simulink model "dec_2_3"  (R2013b)
settings: Solver=ode45  StartTime=0.0  StopTime=10000  RelTol=1e-3
undefined symbols (not defined in the file or in its folder): pfb_coeff_gen_calc, xlfda_numerator, xlipgetpartsetting
libraries: xbsIndex_r4 x2069, casper_library_delays x25, dspsigops x16, casper_library_misc x11, simulink x1, xps_library x1
(part 3 of 19)

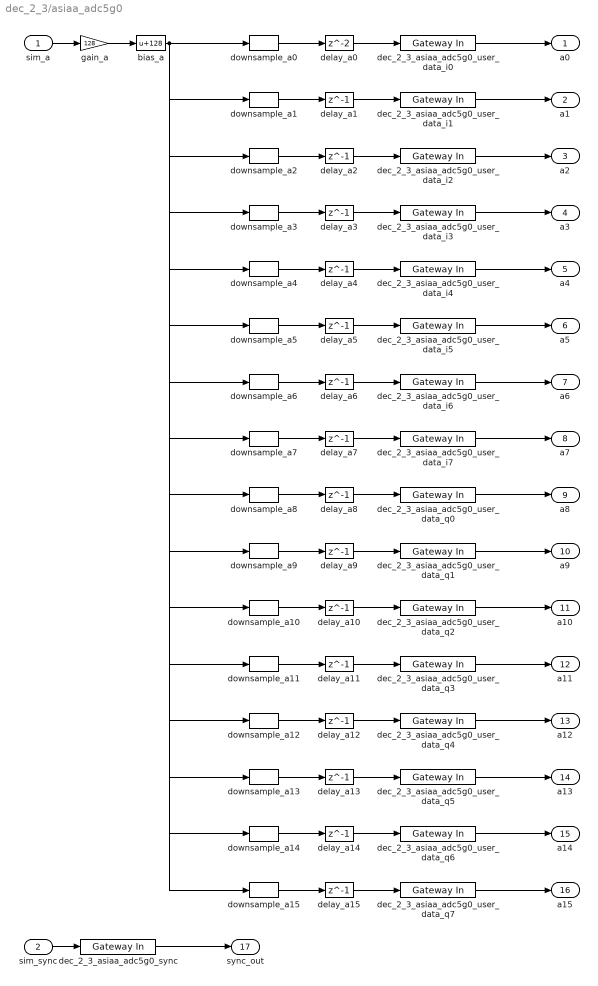
== system dec_2_3/asiaa_adc5g0 ==
  sim_a : Inport
  sim_sync : Inport  Port=2
  bias_a : Bias  Bias=128  SaturateOnIntegerOverflow=on
  dec_2_3_asiaa_adc5g0_sync : xbsIndex_r4/Gateway In  gui_display_data_type=Fixed-point  arith_type=Boolean  n_bits=16  bin_pt=14  preci_type=Single  exp_width=8  frac_width=24  quantization="Round  (unbiased: +/- Inf)"  overflow=Saturate  period=1  dbl_ovrd=off  timing_constraint=None  locs_specified=off  LOCs={}  UseAsADC=off  ADCChannel='1'  inherit_from_input=off  hdl_port=on  block_type=gatewayin
  dec_2_3_asiaa_adc5g0_user_data_i{0..7} (8 alike) : xbsIndex_r4/Gateway In  gui_display_data_type=Fixed-point  arith_type=Unsigned  n_bits=8  bin_pt=0  preci_type=Single  exp_width=8  frac_width=24  quantization=Truncate  overflow=Wrap  period=1  dbl_ovrd=off  timing_constraint=None  locs_specified=off  LOCs={}  UseAsADC=off  ADCChannel='1'  inherit_from_input=off  hdl_port=on  block_type=gatewayin
  dec_2_3_asiaa_adc5g0_user_data_q{0..7} (8 alike) : xbsIndex_r4/Gateway In  gui_display_data_type=Fixed-point  arith_type=Unsigned  n_bits=8  bin_pt=0  preci_type=Single  exp_width=8  frac_width=24  quantization=Truncate  overflow=Wrap  period=1  dbl_ovrd=off  timing_constraint=None  locs_specified=off  LOCs={}  UseAsADC=off  ADCChannel='1'  inherit_from_input=off  hdl_port=on  block_type=gatewayin
  delay_a0 : Delay  InitialCondition=0  InputProcessing=Inherited
  delay_a{1..15} (15 alike) : Delay  DelayLength=1  InitialCondition=0  InputProcessing=Inherited
  downsample_a0 : dspsigops/Downsample  N=16  phase=0  RateOptions=Allow multirate processing  smode=Allow multirate  fmode=Maintain input frame size  ic=0
  downsample_a1 : dspsigops/Downsample  N=16  phase=1  RateOptions=Allow multirate processing  smode=Allow multirate  fmode=Maintain input frame size  ic=0
  downsample_a10 : dspsigops/Downsample  N=16  phase=10  RateOptions=Allow multirate processing  smode=Allow multirate  fmode=Maintain input frame size  ic=0
  downsample_a11 : dspsigops/Downsample  N=16  phase=11  RateOptions=Allow multirate processing  smode=Allow multirate  fmode=Maintain input frame size  ic=0
  downsample_a12 : dspsigops/Downsample  N=16  phase=12  RateOptions=Allow multirate processing  smode=Allow multirate  fmode=Maintain input frame size  ic=0
  downsample_a13 : dspsigops/Downsample  N=16  phase=13  RateOptions=Allow multirate processing  smode=Allow multirate  fmode=Maintain input frame size  ic=0
  downsample_a14 : dspsigops/Downsample  N=16  phase=14  RateOptions=Allow multirate processing  smode=Allow multirate  fmode=Maintain input frame size  ic=0
  downsample_a15 : dspsigops/Downsample  N=16  phase=15  RateOptions=Allow multirate processing  smode=Allow multirate  fmode=Maintain input frame size  ic=0
  downsample_a2 : dspsigops/Downsample  N=16  phase=2  RateOptions=Allow multirate processing  smode=Allow multirate  fmode=Maintain input frame size  ic=0
  downsample_a3 : dspsigops/Downsample  N=16  phase=3  RateOptions=Allow multirate processing  smode=Allow multirate  fmode=Maintain input frame size  ic=0
  downsample_a4 : dspsigops/Downsample  N=16  phase=4  RateOptions=Allow multirate processing  smode=Allow multirate  fmode=Maintain input frame size  ic=0
  downsample_a5 : dspsigops/Downsample  N=16  phase=5  RateOptions=Allow multirate processing  smode=Allow multirate  fmode=Maintain input frame size  ic=0
  downsample_a6 : dspsigops/Downsample  N=16  phase=6  RateOptions=Allow multirate processing  smode=Allow multirate  fmode=Maintain input frame size  ic=0
  downsample_a7 : dspsigops/Downsample  N=16  phase=7  RateOptions=Allow multirate processing  smode=Allow multirate  fmode=Maintain input frame size  ic=0
  downsample_a8 : dspsigops/Downsample  N=16  phase=8  RateOptions=Allow multirate processing  smode=Allow multirate  fmode=Maintain input frame size  ic=0
  downsample_a9 : dspsigops/Downsample  N=16  phase=9  RateOptions=Allow multirate processing  smode=Allow multirate  fmode=Maintain input frame size  ic=0
  gain_a : Gain  Gain=128  SaturateOnIntegerOverflow=on  OutDataTypeStr=Inherit: Same as input  ParamDataTypeStr=Inherit: Same as input
  a0 : Outport
  a1 : Outport  Port=2
  a2 : Outport  Port=3
  a3 : Outport  Port=4
  a4 : Outport  Port=5
  a5 : Outport  Port=6
  a6 : Outport  Port=7
  a7 : Outport  Port=8
  a8 : Outport  Port=9
  a9 : Outport  Port=10
  a10 : Outport  Port=11
  a11 : Outport  Port=12
  a12 : Outport  Port=13
  a13 : Outport  Port=14
  a14 : Outport  Port=15
  a15 : Outport  Port=16
  sync_out : Outport  Port=17
  wires:
  sim_a/1 -> gain_a/1
  gain_a/1 -> bias_a/1
  bias_a/1 -> downsample_a0/1, downsample_a1/1, downsample_a2/1, downsample_a3/1, downsample_a4/1, downsample_a5/1, downsample_a6/1, downsample_a7/1, downsample_a8/1, downsample_a9/1, downsample_a10/1, downsample_a11/1, downsample_a12/1, downsample_a13/1, downsample_a14/1, downsample_a15/1
  downsample_a0/1 -> delay_a0/1
  delay_a0/1 -> dec_2_3_asiaa_adc5g0_user_data_i0/1
  dec_2_3_asiaa_adc5g0_user_data_i0/1 -> a0/1
  downsample_a1/1 -> delay_a1/1
  delay_a1/1 -> dec_2_3_asiaa_adc5g0_user_data_i1/1
  dec_2_3_asiaa_adc5g0_user_data_i1/1 -> a1/1
  downsample_a2/1 -> delay_a2/1
  delay_a2/1 -> dec_2_3_asiaa_adc5g0_user_data_i2/1
  dec_2_3_asiaa_adc5g0_user_data_i2/1 -> a2/1
  downsample_a3/1 -> delay_a3/1
  delay_a3/1 -> dec_2_3_asiaa_adc5g0_user_data_i3/1
  dec_2_3_asiaa_adc5g0_user_data_i3/1 -> a3/1
  downsample_a4/1 -> delay_a4/1
  delay_a4/1 -> dec_2_3_asiaa_adc5g0_user_data_i4/1
  dec_2_3_asiaa_adc5g0_user_data_i4/1 -> a4/1
  downsample_a5/1 -> delay_a5/1
  delay_a5/1 -> dec_2_3_asiaa_adc5g0_user_data_i5/1
  dec_2_3_asiaa_adc5g0_user_data_i5/1 -> a5/1
  downsample_a6/1 -> delay_a6/1
  delay_a6/1 -> dec_2_3_asiaa_adc5g0_user_data_i6/1
  dec_2_3_asiaa_adc5g0_user_data_i6/1 -> a6/1
  downsample_a7/1 -> delay_a7/1
  delay_a7/1 -> dec_2_3_asiaa_adc5g0_user_data_i7/1
  dec_2_3_asiaa_adc5g0_user_data_i7/1 -> a7/1
  downsample_a8/1 -> delay_a8/1
  delay_a8/1 -> dec_2_3_asiaa_adc5g0_user_data_q0/1
  dec_2_3_asiaa_adc5g0_user_data_q0/1 -> a8/1
  downsample_a9/1 -> delay_a9/1
  delay_a9/1 -> dec_2_3_asiaa_adc5g0_user_data_q1/1
  dec_2_3_asiaa_adc5g0_user_data_q1/1 -> a9/1
  downsample_a10/1 -> delay_a10/1
  delay_a10/1 -> dec_2_3_asiaa_adc5g0_user_data_q2/1
  dec_2_3_asiaa_adc5g0_user_data_q2/1 -> a10/1
  downsample_a11/1 -> delay_a11/1
  delay_a11/1 -> dec_2_3_asiaa_adc5g0_user_data_q3/1
  dec_2_3_asiaa_adc5g0_user_data_q3/1 -> a11/1
  downsample_a12/1 -> delay_a12/1
  delay_a12/1 -> dec_2_3_asiaa_adc5g0_user_data_q4/1
  dec_2_3_asiaa_adc5g0_user_data_q4/1 -> a12/1
  downsample_a13/1 -> delay_a13/1
  delay_a13/1 -> dec_2_3_asiaa_adc5g0_user_data_q5/1
  dec_2_3_asiaa_adc5g0_user_data_q5/1 -> a13/1
  downsample_a14/1 -> delay_a14/1
  delay_a14/1 -> dec_2_3_asiaa_adc5g0_user_data_q6/1
  dec_2_3_asiaa_adc5g0_user_data_q6/1 -> a14/1
  downsample_a15/1 -> delay_a15/1
  delay_a15/1 -> dec_2_3_asiaa_adc5g0_user_data_q7/1
  dec_2_3_asiaa_adc5g0_user_data_q7/1 -> a15/1
  sim_sync/1 -> dec_2_3_asiaa_adc5g0_sync/1
  dec_2_3_asiaa_adc5g0_sync/1 -> sync_out/1

== system dec_2_3/bus_create ==
  in1 : Inport
  in2 : Inport  Port=2
  in3 : Inport  Port=3
  in4 : Inport  Port=4
  in5 : Inport  Port=5
  in6 : Inport  Port=6
  in7 : Inport  Port=7
  in8 : Inport  Port=8
  in9 : Inport  Port=9
  in10 : Inport  Port=10
  in11 : Inport  Port=11
  in12 : Inport  Port=12
  in13 : Inport  Port=13
  in14 : Inport  Port=14
  in15 : Inport  Port=15
  in16 : Inport  Port=16
  concatenate : xbsIndex_r4/Concat  num_inputs=16  dbl_ovrd=off  block_type=concat
  reinterpret{1..16} (16 alike) : xbsIndex_r4/Reinterpret  force_arith_type=on  arith_type=Unsigned  force_bin_pt=on  bin_pt=0  block_type=reinterpret
      reinterpret1 settings: infoedit="Changes signal type without altering the binary representation.   You can changed the signal between signed and unsigned, and relocate the binary point.<br><br>Hardware notes: In hardware this block costs nothing.<br><br>Example:  Suppose the input is 6 bits wide, signed, with 2 fractional bits, and the output is forced to unsigned with 0 fractional bits.  Then an input of -2.0 (1110.00 in binary 2's complement) becomes an output of 56 (111000 in binary)."
      reinterpret2 settings: infoedit="Changes signal type without altering the binary representation.   You can changed the signal between signed and unsigned, and relocate the binary point.<br><br>Hardware notes: In hardware this block costs nothing.<br><br>Example:  Suppose the input is 6 bits wide, signed, with 2 fractional bits, and the output is forced to unsigned with 0 fractional bits.  Then an input of -2.0 (1110.00 in binary 2's complement) becomes an output of 56 (111000 in binary)."
  bus_out : Outport
  wires:
  concatenate/1 -> bus_out/1
  in1/1 -> reinterpret1/1
  reinterpret1/1 -> concatenate/1
  in2/1 -> reinterpret2/1
  reinterpret2/1 -> concatenate/2
  in3/1 -> reinterpret3/1
  reinterpret3/1 -> concatenate/3
  in4/1 -> reinterpret4/1
  reinterpret4/1 -> concatenate/4
  in5/1 -> reinterpret5/1
  reinterpret5/1 -> concatenate/5
  in6/1 -> reinterpret6/1
  reinterpret6/1 -> concatenate/6
  in7/1 -> reinterpret7/1
  reinterpret7/1 -> concatenate/7
  in8/1 -> reinterpret8/1
  reinterpret8/1 -> concatenate/8
  in9/1 -> reinterpret9/1
  reinterpret9/1 -> concatenate/9
  in10/1 -> reinterpret10/1
  reinterpret10/1 -> concatenate/10
  in11/1 -> reinterpret11/1
  reinterpret11/1 -> concatenate/11
  in12/1 -> reinterpret12/1
  reinterpret12/1 -> concatenate/12
  in13/1 -> reinterpret13/1
  reinterpret13/1 -> concatenate/13
  in14/1 -> reinterpret14/1
  reinterpret14/1 -> concatenate/14
  in15/1 -> reinterpret15/1
  reinterpret15/1 -> concatenate/15
  in16/1 -> reinterpret16/1
  reinterpret16/1 -> concatenate/16

== system dec_2_3/cnt_rst ==
  dec_2_3_cnt_rst_user_data_out : xbsIndex_r4/Gateway In  gui_display_data_type=Fixed-point  arith_type=Unsigned  n_bits=32  bin_pt=0  preci_type=Single  exp_width=8  frac_width=24  quantization="Round  (unbiased: +/- Inf)"  overflow=Saturate  period=1  dbl_ovrd=off  timing_constraint=None  locs_specified=off  LOCs={}  UseAsADC=off  ADCChannel='1'  inherit_from_input=off  hdl_port=on  block_type=gatewayin
  io_delay : xbsIndex_r4/Delay  rst=off  infoeditControl=Selection of Reset will increase slice count due to use of real FFs and instead of SRLs  en=off  latency=0  dbl_ovrd=off  reg_retiming=on  block_type=delay
  sim_1 : Constant  Value=0
  slice_reg : xbsIndex_r4/Slice  nbits=32  boolean_output=on  mode=Lower Bit Location + Width  bit1=0  base1=MSB of Input  bit0=0  base0=LSB of Input  dbl_ovrd=off  block_type=slice
  in_reg : Outport
  wires:
  dec_2_3_cnt_rst_user_data_out/1 -> io_delay/1
  sim_1/1 -> dec_2_3_cnt_rst_user_data_out/1
  io_delay/1 -> slice_reg/1
  slice_reg/1 -> in_reg/1

== system dec_2_3/conv_bus0 ==
  i0 : Inport
  i1 : Inport  Port=2
  i2 : Inport  Port=3
  i3 : Inport  Port=4
  i4 : Inport  Port=5
  i5 : Inport  Port=6
  i6 : Inport  Port=7
  i7 : Inport  Port=8
  i8 : Inport  Port=9
  i9 : Inport  Port=10
  i10 : Inport  Port=11
  i11 : Inport  Port=12
  i12 : Inport  Port=13
  i13 : Inport  Port=14
  i14 : Inport  Port=15
  i15 : Inport  Port=16
  conv_ob0 : Subsystem
  conv_ob1 : Subsystem
  conv_ob10 : Subsystem
  conv_ob11 : Subsystem
  conv_ob12 : Subsystem
  conv_ob13 : Subsystem
  conv_ob14 : Subsystem
  conv_ob15 : Subsystem
  conv_ob2 : Subsystem
  conv_ob3 : Subsystem
  conv_ob4 : Subsystem
  conv_ob5 : Subsystem
  conv_ob6 : Subsystem
  conv_ob7 : Subsystem
  conv_ob8 : Subsystem
  conv_ob9 : Subsystem
  q0 : Outport
  q1 : Outport  Port=2
  q2 : Outport  Port=3
  q3 : Outport  Port=4
  q4 : Outport  Port=5
  q5 : Outport  Port=6
  q6 : Outport  Port=7
  q7 : Outport  Port=8
  q8 : Outport  Port=9
  q9 : Outport  Port=10
  q10 : Outport  Port=11
  q11 : Outport  Port=12
  q12 : Outport  Port=13
  q13 : Outport  Port=14
  q14 : Outport  Port=15
  q15 : Outport  Port=16
  wires:
  conv_ob7/1(q) -> q7/1
  i7/1 -> conv_ob7/1(i)
  conv_ob6/1(q) -> q6/1
  i6/1 -> conv_ob6/1(i)
  conv_ob5/1(q) -> q5/1
  i5/1 -> conv_ob5/1(i)
  conv_ob4/1(q) -> q4/1
  i4/1 -> conv_ob4/1(i)
  conv_ob3/1(q) -> q3/1
  i3/1 -> conv_ob3/1(i)
  conv_ob2/1(q) -> q2/1
  i2/1 -> conv_ob2/1(i)
  conv_ob1/1(q) -> q1/1
  i1/1 -> conv_ob1/1(i)
  conv_ob0/1(q) -> q0/1
  i0/1 -> conv_ob0/1(i)
  conv_ob15/1(q) -> q15/1
  i15/1 -> conv_ob15/1(i)
  conv_ob14/1(q) -> q14/1
  i14/1 -> conv_ob14/1(i)
  conv_ob13/1(q) -> q13/1
  i13/1 -> conv_ob13/1(i)
  conv_ob12/1(q) -> q12/1
  i12/1 -> conv_ob12/1(i)
  conv_ob11/1(q) -> q11/1
  i11/1 -> conv_ob11/1(i)
  conv_ob10/1(q) -> q10/1
  i10/1 -> conv_ob10/1(i)
  conv_ob9/1(q) -> q9/1
  i9/1 -> conv_ob9/1(i)
  conv_ob8/1(q) -> q8/1
  i8/1 -> conv_ob8/1(i)

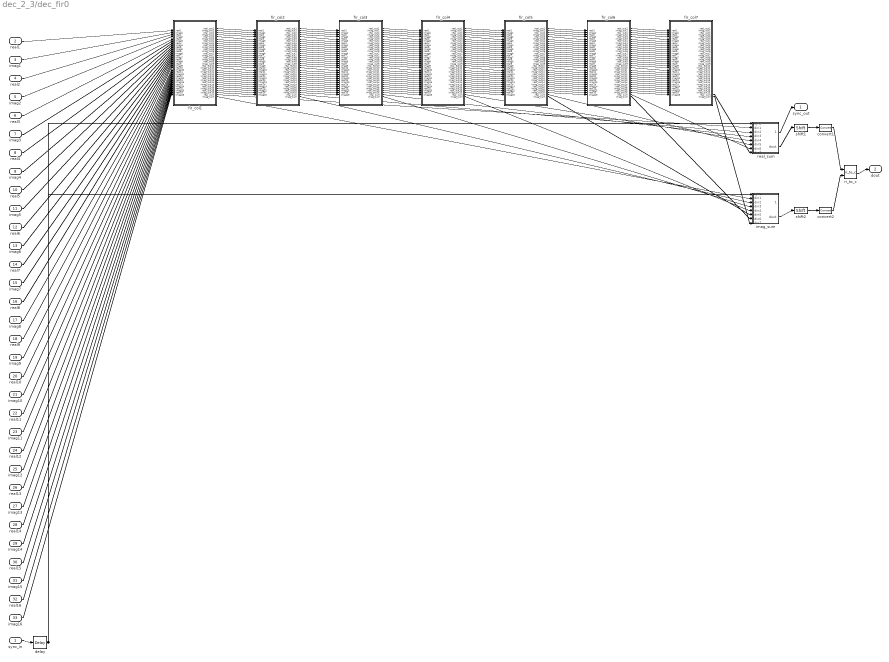
== system dec_2_3/dec_fir0 ==
  sync_in : Inport
  real1 : Inport  Port=2
  imag1 : Inport  Port=3
  real2 : Inport  Port=4
  imag2 : Inport  Port=5
  real3 : Inport  Port=6
  imag3 : Inport  Port=7
  real4 : Inport  Port=8
  imag4 : Inport  Port=9
  real5 : Inport  Port=10
  imag5 : Inport  Port=11
  real6 : Inport  Port=12
  imag6 : Inport  Port=13
  real7 : Inport  Port=14
  imag7 : Inport  Port=15
  real8 : Inport  Port=16
  imag8 : Inport  Port=17
  real9 : Inport  Port=18
  imag9 : Inport  Port=19
  real10 : Inport  Port=20
  imag10 : Inport  Port=21
  real11 : Inport  Port=22
  imag11 : Inport  Port=23
  real12 : Inport  Port=24
  imag12 : Inport  Port=25
  real13 : Inport  Port=26
  imag13 : Inport  Port=27
  real14 : Inport  Port=28
  imag14 : Inport  Port=29
  real15 : Inport  Port=30
  imag15 : Inport  Port=31
  real16 : Inport  Port=32
  imag16 : Inport  Port=33
  convert1 : xbsIndex_r4/Convert  gui_display_data_type=Fixed-point  arith_type="Signed  (2's comp)"  n_bits=30  bin_pt=29  float_type=Single  exp_bits=8  fraction_bits=24  quantization="Round  (unbiased: +/- Inf)"  overflow=Wrap  en=off  latency=2  dbl_ovrd=off  pipeline=off  block_type=convert
  convert2 : xbsIndex_r4/Convert  gui_display_data_type=Fixed-point  arith_type="Signed  (2's comp)"  n_bits=30  bin_pt=29  float_type=Single  exp_bits=8  fraction_bits=24  quantization="Round  (unbiased: +/- Inf)"  overflow=Wrap  en=off  latency=2  dbl_ovrd=off  pipeline=off  block_type=convert
  delay : xbsIndex_r4/Delay  rst=off  infoeditControl=Selection of Reset will increase slice count due to use of real FFs and instead of SRLs  en=off  latency=8  dbl_ovrd=off  reg_retiming=off  block_type=delay
  fir_col1 : Subsystem  AncestorBlock=casper_library_downconverter/fir_col  mask(fir_col){n_inputs=16, coeff=[0.0062127   0.0053266   0.0042757   0.0031122     0.00189  0.00066203 -0.00052147   -0.001615  -0.0025791  -0.0033818  -0.0039996  -0.0044174  -0.0046295  -0.0046386  -0.0044554  -0.0040983], add_latency=1, mult_latency=2, coeff_bit_width=25, coeff_bin_pt=24, first_stage_hdl=on, adder_imp=DSP48}
      mask prompts: n_inputs "Inputs"; coeff "Coefficients"; add_latency "Add latency"; mult_latency "Mult Latency"; coeff_bit_width "Coefficient bit width"; coeff_bin_pt "Coefficient binary point"; first_stage_hdl "Implement first stage of adder trees on output as behavioural HDL"; adder_imp "Adder implementation"
      mask init:
      | fir_col_init(gcb, ...
      |     'n_inputs', n_inputs,...
      |     'coeff', coeff, ...
      |     'mult_latency', mult_latency, ...
      |     'add_latency', add_latency, ...
      |     'coeff_bit_width', coeff_bit_width, ...
      |     'coeff_bin_pt', coeff_bin_pt, ...
      |     'first_stage_hdl', first_stage_hdl, ...
      |     'adder_imp', adder_imp);
      mask Help: eval('xlWeb(''http://casper.berkeley.edu/wiki/Fir_col'')')
      mask TypeOptions adder_imp: Behavioral | Fabric | DSP48
  fir_col2 : Subsystem  AncestorBlock=casper_library_downconverter/fir_col  mask(fir_col){n_inputs=16, coeff=[-0.011813   -0.010354  -0.0085971  -0.0066339  -0.0045559   -0.002452 -0.00040564   0.0015077   0.0032228   0.0046863    0.005858   0.0067112   0.0072334   0.0074255    0.007301   0.0068851], add_latency=1, mult_latency=2, coeff_bit_width=25, coeff_bin_pt=24, first_stage_hdl=on, adder_imp=DSP48}
      mask prompts: n_inputs "Inputs"; coeff "Coefficients"; add_latency "Add latency"; mult_latency "Mult Latency"; coeff_bit_width "Coefficient bit width"; coeff_bin_pt "Coefficient binary point"; first_stage_hdl "Implement first stage of adder trees on output as behavioural HDL"; adder_imp "Adder implementation"
      mask init: same as dec_2_3/dec_fir0/fir_col1
      mask Help: eval('xlWeb(''http://casper.berkeley.edu/wiki/Fir_col'')')
      mask TypeOptions adder_imp: Behavioral | Fabric | DSP48
  fir_col3 : Subsystem  AncestorBlock=casper_library_downconverter/fir_col  mask(fir_col){n_inputs=16, coeff=[0.036703    0.030974     0.02517    0.019424    0.013861   0.0086017   0.0037501 -0.00060339   -0.004386  -0.0075441   -0.010044   -0.011873   -0.013038   -0.013563   -0.013493   -0.012886], add_latency=1, mult_latency=2, coeff_bit_width=25, coeff_bin_pt=24, first_stage_hdl=on, adder_imp=DSP48}
      mask prompts: n_inputs "Inputs"; coeff "Coefficients"; add_latency "Add latency"; mult_latency "Mult Latency"; coeff_bit_width "Coefficient bit width"; coeff_bin_pt "Coefficient binary point"; first_stage_hdl "Implement first stage of adder trees on output as behavioural HDL"; adder_imp "Adder implementation"
      mask init: same as dec_2_3/dec_fir0/fir_col1
      mask Help: eval('xlWeb(''http://casper.berkeley.edu/wiki/Fir_col'')')
      mask TypeOptions adder_imp: Behavioral | Fabric | DSP48
  fir_col4 : Subsystem  AncestorBlock=casper_library_downconverter/fir_col  mask(fir_col){n_inputs=16, coeff=[0.042221    0.047395      0.0521    0.056218    0.059645    0.062295    0.064101    0.065015    0.065015    0.064101    0.062295    0.059645    0.056218      0.0521    0.047395    0.042221], add_latency=1, mult_latency=2, coeff_bit_width=25, coeff_bin_pt=24, first_stage_hdl=on, adder_imp=DSP48}
      mask prompts: n_inputs "Inputs"; coeff "Coefficients"; add_latency "Add latency"; mult_latency "Mult Latency"; coeff_bit_width "Coefficient bit width"; coeff_bin_pt "Coefficient binary point"; first_stage_hdl "Implement first stage of adder trees on output as behavioural HDL"; adder_imp "Adder implementation"
      mask init: same as dec_2_3/dec_fir0/fir_col1
      mask Help: eval('xlWeb(''http://casper.berkeley.edu/wiki/Fir_col'')')
      mask TypeOptions adder_imp: Behavioral | Fabric | DSP48
  fir_col5 : Subsystem  AncestorBlock=casper_library_downconverter/fir_col  mask(fir_col){n_inputs=16, coeff=[-0.012886   -0.013493   -0.013563   -0.013038   -0.011873   -0.010044  -0.0075441   -0.004386 -0.00060339   0.0037501   0.0086017    0.013861    0.019424     0.02517    0.030974    0.036703], add_latency=1, mult_latency=2, coeff_bit_width=25, coeff_bin_pt=24, first_stage_hdl=on, adder_imp=DSP48}
      mask prompts: n_inputs "Inputs"; coeff "Coefficients"; add_latency "Add latency"; mult_latency "Mult Latency"; coeff_bit_width "Coefficient bit width"; coeff_bin_pt "Coefficient binary point"; first_stage_hdl "Implement first stage of adder trees on output as behavioural HDL"; adder_imp "Adder implementation"
      mask init: same as dec_2_3/dec_fir0/fir_col1
      mask Help: eval('xlWeb(''http://casper.berkeley.edu/wiki/Fir_col'')')
      mask TypeOptions adder_imp: Behavioral | Fabric | DSP48
  fir_col6 : Subsystem  AncestorBlock=casper_library_downconverter/fir_col  mask(fir_col){n_inputs=16, coeff=[0.0068851    0.007301   0.0074255   0.0072334   0.0067112    0.005858   0.0046863   0.0032228   0.0015077 -0.00040564   -0.002452  -0.0045559  -0.0066339  -0.0085971   -0.010354   -0.011813], add_latency=1, mult_latency=2, coeff_bit_width=25, coeff_bin_pt=24, first_stage_hdl=on, adder_imp=DSP48}
      mask prompts: n_inputs "Inputs"; coeff "Coefficients"; add_latency "Add latency"; mult_latency "Mult Latency"; coeff_bit_width "Coefficient bit width"; coeff_bin_pt "Coefficient binary point"; first_stage_hdl "Implement first stage of adder trees on output as behavioural HDL"; adder_imp "Adder implementation"
      mask init: same as dec_2_3/dec_fir0/fir_col1
      mask Help: eval('xlWeb(''http://casper.berkeley.edu/wiki/Fir_col'')')
      mask TypeOptions adder_imp: Behavioral | Fabric | DSP48
  fir_col7 : Subsystem  AncestorBlock=casper_library_downconverter/fir_col  mask(fir_col){n_inputs=16, coeff=[-0.0040983  -0.0044554  -0.0046386  -0.0046295  -0.0044174  -0.0039996  -0.0033818  -0.0025791   -0.001615 -0.00052147  0.00066203     0.00189   0.0031122   0.0042757   0.0053266   0.0062127], add_latency=1, mult_latency=2, coeff_bit_width=25, coeff_bin_pt=24, first_stage_hdl=on, adder_imp=DSP48}
      mask prompts: n_inputs "Inputs"; coeff "Coefficients"; add_latency "Add latency"; mult_latency "Mult Latency"; coeff_bit_width "Coefficient bit width"; coeff_bin_pt "Coefficient binary point"; first_stage_hdl "Implement first stage of adder trees on output as behavioural HDL"; adder_imp "Adder implementation"
      mask init: same as dec_2_3/dec_fir0/fir_col1
      mask Help: eval('xlWeb(''http://casper.berkeley.edu/wiki/Fir_col'')')
      mask TypeOptions adder_imp: Behavioral | Fabric | DSP48
  imag_sum : Subsystem  AncestorBlock=casper_library_misc/adder_tree  mask(adder_tree){n_inputs=7, latency=1, adder_imp=DSP48, first_stage_hdl=off}
      mask prompts: n_inputs "Number of Inputs"; latency "Add Latency"; adder_imp "Adder implementation"; first_stage_hdl "Use behavioural HDL for first stage of adders"
      mask help:
      | Sums all inputs using a tree of adds and delays.
      |
      | Number of inputs: The number of inputs to the block to be summed
      | Add latency: The number of clock cycles to perform one addition (affects timing)..
      | Adder implementation: choice of fabric or DSP48E core, or behavioral HDL
      | Use behavioural HDL for first stage of adders: Causes the first stage of adders to be absorbed into DSP blocks if multipliers precede them (Virtex 5). Overrides Adder implementation
      mask init:
      | adder_tree_init(gcb, ...
      |     'n_inputs', n_inputs, ...
      |     'latency', latency, ...
      |     'adder_imp', adder_imp, ...
      |     'first_stage_hdl', first_stage_hdl);
      settings: AttributesFormatString=latency 3
      mask Help: eval('xlWeb(''http://casper.berkeley.edu/wiki/Adder_tree'')')
      mask TypeOptions adder_imp: Behavioral | Fabric | DSP48
  real_sum : Subsystem  AncestorBlock=casper_library_misc/adder_tree  mask(adder_tree){n_inputs=7, latency=1, adder_imp=DSP48, first_stage_hdl=off}
      mask prompts: n_inputs "Number of Inputs"; latency "Add Latency"; adder_imp "Adder implementation"; first_stage_hdl "Use behavioural HDL for first stage of adders"
      mask help:
      | Sums all inputs using a tree of adds and delays.
      |
      | Number of inputs: The number of inputs to the block to be summed
      | Add latency: The number of clock cycles to perform one addition (affects timing)..
      | Adder implementation: choice of fabric or DSP48E core, or behavioral HDL
      | Use behavioural HDL for first stage of adders: Causes the first stage of adders to be absorbed into DSP blocks if multipliers precede them (Virtex 5). Overrides Adder implementation
      mask init:
      | adder_tree_init(gcb, ...
      |     'n_inputs', n_inputs, ...
      |     'latency', latency, ...
      |     'adder_imp', adder_imp, ...
      |     'first_stage_hdl', first_stage_hdl);
      settings: AttributesFormatString=latency 3
      mask Help: eval('xlWeb(''http://casper.berkeley.edu/wiki/Adder_tree'')')
      mask TypeOptions adder_imp: Behavioral | Fabric | DSP48
  ri_to_c : casper_library_misc/ri_to_c
  shift1 : xbsIndex_r4/Shift  shift_dir=Left  shift_bits=0  en=off  latency=0  precision=Full  arith_type="Signed  (2's comp)"  n_bits=16  bin_pt=14  quantization=Truncate  overflow=Wrap  dbl_ovrd=off  block_type=shift
  shift2 : xbsIndex_r4/Shift  shift_dir=Left  shift_bits=0  en=off  latency=0  precision=Full  arith_type="Signed  (2's comp)"  n_bits=16  bin_pt=14  quantization=Truncate  overflow=Wrap  dbl_ovrd=off  block_type=shift
  sync_out : Outport
  dout : Outport  Port=2
  wires:
  real1/1 -> fir_col1/1(real1)
  imag1/1 -> fir_col1/2(imag1)
  real2/1 -> fir_col1/3(real2)
  imag2/1 -> fir_col1/4(imag2)
  real3/1 -> fir_col1/5(real3)
  imag3/1 -> fir_col1/6(imag3)
  real4/1 -> fir_col1/7(real4)
  imag4/1 -> fir_col1/8(imag4)
  real5/1 -> fir_col1/9(real5)
  imag5/1 -> fir_col1/10(imag5)
  real6/1 -> fir_col1/11(real6)
  imag6/1 -> fir_col1/12(imag6)
  real7/1 -> fir_col1/13(real7)
  imag7/1 -> fir_col1/14(imag7)
  real8/1 -> fir_col1/15(real8)
  imag8/1 -> fir_col1/16(imag8)
  real9/1 -> fir_col1/17(real9)
  imag9/1 -> fir_col1/18(imag9)
  real10/1 -> fir_col1/19(real10)
  imag10/1 -> fir_col1/20(imag10)
  real11/1 -> fir_col1/21(real11)
  imag11/1 -> fir_col1/22(imag11)
  real12/1 -> fir_col1/23(real12)
  imag12/1 -> fir_col1/24(imag12)
  real13/1 -> fir_col1/25(real13)
  imag13/1 -> fir_col1/26(imag13)
  real14/1 -> fir_col1/27(real14)
  imag14/1 -> fir_col1/28(imag14)
  real15/1 -> fir_col1/29(real15)
  imag15/1 -> fir_col1/30(imag15)
  real16/1 -> fir_col1/31(real16)
  imag16/1 -> fir_col1/32(imag16)
  fir_col1/33(real_sum) -> real_sum/2(din1)
  fir_col1/34(imag_sum) -> imag_sum/2(din1)
  fir_col1/1(real_out1) -> fir_col2/1(real1)
  fir_col1/2(imag_out1) -> fir_col2/2(imag1)
  fir_col1/3(real_out2) -> fir_col2/3(real2)
  fir_col1/4(imag_out2) -> fir_col2/4(imag2)
  fir_col1/5(real_out3) -> fir_col2/5(real3)
  fir_col1/6(imag_out3) -> fir_col2/6(imag3)
  fir_col1/7(real_out4) -> fir_col2/7(real4)
  fir_col1/8(imag_out4) -> fir_col2/8(imag4)
  fir_col1/9(real_out5) -> fir_col2/9(real5)
  fir_col1/10(imag_out5) -> fir_col2/10(imag5)
  fir_col1/11(real_out6) -> fir_col2/11(real6)
  fir_col1/12(imag_out6) -> fir_col2/12(imag6)
  fir_col1/13(real_out7) -> fir_col2/13(real7)
  fir_col1/14(imag_out7) -> fir_col2/14(imag7)
  fir_col1/15(real_out8) -> fir_col2/15(real8)
  fir_col1/16(imag_out8) -> fir_col2/16(imag8)
  fir_col1/17(real_out9) -> fir_col2/17(real9)
  fir_col1/18(imag_out9) -> fir_col2/18(imag9)
  fir_col1/19(real_out10) -> fir_col2/19(real10)
  fir_col1/20(imag_out10) -> fir_col2/20(imag10)
  fir_col1/21(real_out11) -> fir_col2/21(real11)
  fir_col1/22(imag_out11) -> fir_col2/22(imag11)
  fir_col1/23(real_out12) -> fir_col2/23(real12)
  fir_col1/24(imag_out12) -> fir_col2/24(imag12)
  fir_col1/25(real_out13) -> fir_col2/25(real13)
  fir_col1/26(imag_out13) -> fir_col2/26(imag13)
  fir_col1/27(real_out14) -> fir_col2/27(real14)
  fir_col1/28(imag_out14) -> fir_col2/28(imag14)
  fir_col1/29(real_out15) -> fir_col2/29(real15)
  fir_col1/30(imag_out15) -> fir_col2/30(imag15)
  fir_col1/31(real_out16) -> fir_col2/31(real16)
  fir_col1/32(imag_out16) -> fir_col2/32(imag16)
  fir_col2/33(real_sum) -> real_sum/3(din2)
  fir_col2/34(imag_sum) -> imag_sum/3(din2)
  fir_col2/1(real_out1) -> fir_col3/1(real1)
  fir_col2/2(imag_out1) -> fir_col3/2(imag1)
  fir_col2/3(real_out2) -> fir_col3/3(real2)
  fir_col2/4(imag_out2) -> fir_col3/4(imag2)
  fir_col2/5(real_out3) -> fir_col3/5(real3)
  fir_col2/6(imag_out3) -> fir_col3/6(imag3)
  fir_col2/7(real_out4) -> fir_col3/7(real4)
  fir_col2/8(imag_out4) -> fir_col3/8(imag4)
  fir_col2/9(real_out5) -> fir_col3/9(real5)
  fir_col2/10(imag_out5) -> fir_col3/10(imag5)
  fir_col2/11(real_out6) -> fir_col3/11(real6)
  fir_col2/12(imag_out6) -> fir_col3/12(imag6)
  fir_col2/13(real_out7) -> fir_col3/13(real7)
  fir_col2/14(imag_out7) -> fir_col3/14(imag7)
  fir_col2/15(real_out8) -> fir_col3/15(real8)
  fir_col2/16(imag_out8) -> fir_col3/16(imag8)
  fir_col2/17(real_out9) -> fir_col3/17(real9)
  fir_col2/18(imag_out9) -> fir_col3/18(imag9)
  fir_col2/19(real_out10) -> fir_col3/19(real10)
  fir_col2/20(imag_out10) -> fir_col3/20(imag10)
  fir_col2/21(real_out11) -> fir_col3/21(real11)
  fir_col2/22(imag_out11) -> fir_col3/22(imag11)
  fir_col2/23(real_out12) -> fir_col3/23(real12)
  fir_col2/24(imag_out12) -> fir_col3/24(imag12)
  fir_col2/25(real_out13) -> fir_col3/25(real13)
  fir_col2/26(imag_out13) -> fir_col3/26(imag13)
  fir_col2/27(real_out14) -> fir_col3/27(real14)
  fir_col2/28(imag_out14) -> fir_col3/28(imag14)
  fir_col2/29(real_out15) -> fir_col3/29(real15)
  fir_col2/30(imag_out15) -> fir_col3/30(imag15)
  fir_col2/31(real_out16) -> fir_col3/31(real16)
  fir_col2/32(imag_out16) -> fir_col3/32(imag16)
  fir_col3/33(real_sum) -> real_sum/4(din3)
  fir_col3/34(imag_sum) -> imag_sum/4(din3)
  fir_col3/1(real_out1) -> fir_col4/1(real1)
  fir_col3/2(imag_out1) -> fir_col4/2(imag1)
  fir_col3/3(real_out2) -> fir_col4/3(real2)
  fir_col3/4(imag_out2) -> fir_col4/4(imag2)
  fir_col3/5(real_out3) -> fir_col4/5(real3)
  fir_col3/6(imag_out3) -> fir_col4/6(imag3)
  fir_col3/7(real_out4) -> fir_col4/7(real4)
  fir_col3/8(imag_out4) -> fir_col4/8(imag4)
  fir_col3/9(real_out5) -> fir_col4/9(real5)
  fir_col3/10(imag_out5) -> fir_col4/10(imag5)
  fir_col3/11(real_out6) -> fir_col4/11(real6)
  fir_col3/12(imag_out6) -> fir_col4/12(imag6)
  fir_col3/13(real_out7) -> fir_col4/13(real7)
  fir_col3/14(imag_out7) -> fir_col4/14(imag7)
  fir_col3/15(real_out8) -> fir_col4/15(real8)
  fir_col3/16(imag_out8) -> fir_col4/16(imag8)
  fir_col3/17(real_out9) -> fir_col4/17(real9)
  fir_col3/18(imag_out9) -> fir_col4/18(imag9)
  fir_col3/19(real_out10) -> fir_col4/19(real10)
  fir_col3/20(imag_out10) -> fir_col4/20(imag10)
  fir_col3/21(real_out11) -> fir_col4/21(real11)
  fir_col3/22(imag_out11) -> fir_col4/22(imag11)
  fir_col3/23(real_out12) -> fir_col4/23(real12)
  fir_col3/24(imag_out12) -> fir_col4/24(imag12)
  fir_col3/25(real_out13) -> fir_col4/25(real13)
  fir_col3/26(imag_out13) -> fir_col4/26(imag13)
  fir_col3/27(real_out14) -> fir_col4/27(real14)
  fir_col3/28(imag_out14) -> fir_col4/28(imag14)
  fir_col3/29(real_out15) -> fir_col4/29(real15)
  fir_col3/30(imag_out15) -> fir_col4/30(imag15)
  fir_col3/31(real_out16) -> fir_col4/31(real16)
  fir_col3/32(imag_out16) -> fir_col4/32(imag16)
  fir_col4/33(real_sum) -> real_sum/5(din4)
  fir_col4/34(imag_sum) -> imag_sum/5(din4)
  fir_col4/1(real_out1) -> fir_col5/1(real1)
  fir_col4/2(imag_out1) -> fir_col5/2(imag1)
  fir_col4/3(real_out2) -> fir_col5/3(real2)
  fir_col4/4(imag_out2) -> fir_col5/4(imag2)
  fir_col4/5(real_out3) -> fir_col5/5(real3)
  fir_col4/6(imag_out3) -> fir_col5/6(imag3)
  fir_col4/7(real_out4) -> fir_col5/7(real4)
  fir_col4/8(imag_out4) -> fir_col5/8(imag4)
  fir_col4/9(real_out5) -> fir_col5/9(real5)
  fir_col4/10(imag_out5) -> fir_col5/10(imag5)
  fir_col4/11(real_out6) -> fir_col5/11(real6)
  fir_col4/12(imag_out6) -> fir_col5/12(imag6)
  fir_col4/13(real_out7) -> fir_col5/13(real7)
  fir_col4/14(imag_out7) -> fir_col5/14(imag7)
  fir_col4/15(real_out8) -> fir_col5/15(real8)
  fir_col4/16(imag_out8) -> fir_col5/16(imag8)
  fir_col4/17(real_out9) -> fir_col5/17(real9)
  fir_col4/18(imag_out9) -> fir_col5/18(imag9)
  fir_col4/19(real_out10) -> fir_col5/19(real10)
  fir_col4/20(imag_out10) -> fir_col5/20(imag10)
  fir_col4/21(real_out11) -> fir_col5/21(real11)
  fir_col4/22(imag_out11) -> fir_col5/22(imag11)
  fir_col4/23(real_out12) -> fir_col5/23(real12)
  fir_col4/24(imag_out12) -> fir_col5/24(imag12)
  fir_col4/25(real_out13) -> fir_col5/25(real13)
  fir_col4/26(imag_out13) -> fir_col5/26(imag13)
  fir_col4/27(real_out14) -> fir_col5/27(real14)
  fir_col4/28(imag_out14) -> fir_col5/28(imag14)
  fir_col4/29(real_out15) -> fir_col5/29(real15)
  fir_col4/30(imag_out15) -> fir_col5/30(imag15)
  fir_col4/31(real_out16) -> fir_col5/31(real16)
  fir_col4/32(imag_out16) -> fir_col5/32(imag16)
  fir_col5/33(real_sum) -> real_sum/6(din5)
  fir_col5/34(imag_sum) -> imag_sum/6(din5)
  fir_col5/1(real_out1) -> fir_col6/1(real1)
  fir_col5/2(imag_out1) -> fir_col6/2(imag1)
  fir_col5/3(real_out2) -> fir_col6/3(real2)
  fir_col5/4(imag_out2) -> fir_col6/4(imag2)
  fir_col5/5(real_out3) -> fir_col6/5(real3)
  fir_col5/6(imag_out3) -> fir_col6/6(imag3)
  fir_col5/7(real_out4) -> fir_col6/7(real4)
  fir_col5/8(imag_out4) -> fir_col6/8(imag4)
  fir_col5/9(real_out5) -> fir_col6/9(real5)
  fir_col5/10(imag_out5) -> fir_col6/10(imag5)
  fir_col5/11(real_out6) -> fir_col6/11(real6)
  fir_col5/12(imag_out6) -> fir_col6/12(imag6)
  fir_col5/13(real_out7) -> fir_col6/13(real7)
  fir_col5/14(imag_out7) -> fir_col6/14(imag7)
  fir_col5/15(real_out8) -> fir_col6/15(real8)
  fir_col5/16(imag_out8) -> fir_col6/16(imag8)
  fir_col5/17(real_out9) -> fir_col6/17(real9)
  fir_col5/18(imag_out9) -> fir_col6/18(imag9)
  fir_col5/19(real_out10) -> fir_col6/19(real10)
  fir_col5/20(imag_out10) -> fir_col6/20(imag10)
  fir_col5/21(real_out11) -> fir_col6/21(real11)
  fir_col5/22(imag_out11) -> fir_col6/22(imag11)
  fir_col5/23(real_out12) -> fir_col6/23(real12)
  fir_col5/24(imag_out12) -> fir_col6/24(imag12)
  fir_col5/25(real_out13) -> fir_col6/25(real13)
  fir_col5/26(imag_out13) -> fir_col6/26(imag13)
  fir_col5/27(real_out14) -> fir_col6/27(real14)
  fir_col5/28(imag_out14) -> fir_col6/28(imag14)
  fir_col5/29(real_out15) -> fir_col6/29(real15)
  fir_col5/30(imag_out15) -> fir_col6/30(imag15)
  fir_col5/31(real_out16) -> fir_col6/31(real16)
  fir_col5/32(imag_out16) -> fir_col6/32(imag16)
  fir_col6/33(real_sum) -> real_sum/7(din6)
  fir_col6/34(imag_sum) -> imag_sum/7(din6)
  fir_col6/1(real_out1) -> fir_col7/1(real1)
  fir_col6/2(imag_out1) -> fir_col7/2(imag1)
  fir_col6/3(real_out2) -> fir_col7/3(real2)
  fir_col6/4(imag_out2) -> fir_col7/4(imag2)
  fir_col6/5(real_out3) -> fir_col7/5(real3)
  fir_col6/6(imag_out3) -> fir_col7/6(imag3)
  fir_col6/7(real_out4) -> fir_col7/7(real4)
  fir_col6/8(imag_out4) -> fir_col7/8(imag4)
  fir_col6/9(real_out5) -> fir_col7/9(real5)
  fir_col6/10(imag_out5) -> fir_col7/10(imag5)
  fir_col6/11(real_out6) -> fir_col7/11(real6)
  fir_col6/12(imag_out6) -> fir_col7/12(imag6)
  fir_col6/13(real_out7) -> fir_col7/13(real7)
  fir_col6/14(imag_out7) -> fir_col7/14(imag7)
  fir_col6/15(real_out8) -> fir_col7/15(real8)
  fir_col6/16(imag_out8) -> fir_col7/16(imag8)
  fir_col6/17(real_out9) -> fir_col7/17(real9)
  fir_col6/18(imag_out9) -> fir_col7/18(imag9)
  fir_col6/19(real_out10) -> fir_col7/19(real10)
  fir_col6/20(imag_out10) -> fir_col7/20(imag10)
  fir_col6/21(real_out11) -> fir_col7/21(real11)
  fir_col6/22(imag_out11) -> fir_col7/22(imag11)
  fir_col6/23(real_out12) -> fir_col7/23(real12)
  fir_col6/24(imag_out12) -> fir_col7/24(imag12)
  fir_col6/25(real_out13) -> fir_col7/25(real13)
  fir_col6/26(imag_out13) -> fir_col7/26(imag13)
  fir_col6/27(real_out14) -> fir_col7/27(real14)
  fir_col6/28(imag_out14) -> fir_col7/28(imag14)
  fir_col6/29(real_out15) -> fir_col7/29(real15)
  fir_col6/30(imag_out15) -> fir_col7/30(imag15)
  fir_col6/31(real_out16) -> fir_col7/31(real16)
  fir_col6/32(imag_out16) -> fir_col7/32(imag16)
  fir_col7/33(real_sum) -> real_sum/8(din7)
  fir_col7/34(imag_sum) -> imag_sum/8(din7)
  real_sum/2(dout) -> shift1/1
  imag_sum/2(dout) -> shift2/1
  shift1/1 -> convert1/1
  shift2/1 -> convert2/1
  convert1/1 -> ri_to_c/1
  convert2/1 -> ri_to_c/2
  ri_to_c/1 -> dout/1
  sync_in/1 -> delay/1
  delay/1 -> real_sum/1(sync), imag_sum/1(sync)
  real_sum/1(sync_out) -> sync_out/1
